simulink model "DAPS_SA_MdlIdent"  (R2017a)
settings: Solver=FixedStepAuto  StartTime=0  StopTime=68  FixedStep=0.001  MaxStep=0.01  RelTol=1e-4
undefined symbols (not defined in the file or in its folder): mdlPara
libraries: PASL_Mechanics x4, PASL_Models x2, PASL_Tools x2, PASL_Pneumatics x2, PASL_Components x1
settings Model: Creator=MMNT  LastModifiedBy=mmnt

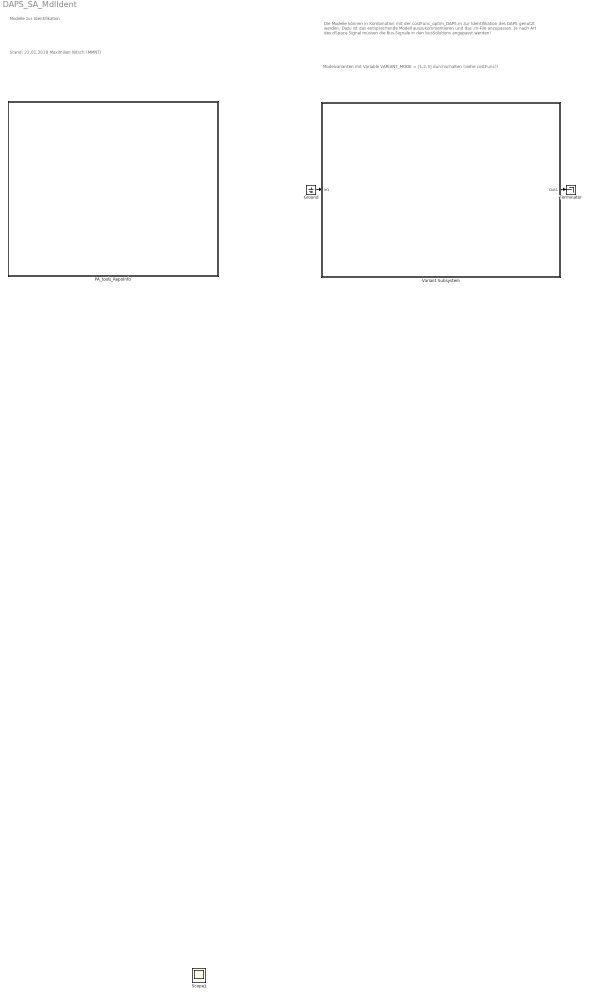
== system DAPS_SA_MdlIdent ==
  note: Modelvarianten mit Variable VARIANT_MODE = [1,2,3] durchschalten (siehe costFunc)!
  note: Die Modelle können in Kombination mit der costFunc_optim_DAPS.m
      | zur Identifikation des DAPS genutzt werden. Dazu ist das entsprechende
      | Modell auszukommentieren und das .m-File anzupassen. Je nach Art des
      | dSpace Signal müssen die Bus-Signale in den busSolutions angepasst werden!
  note: Modelle zur Identifikation
  note: Stand: 22.01.2018
      | Maximilian Nitsch (MMNT)
  Ground : Ground
  PA_tools_RepoInfo : Subsystem  Tag=RevTagSubSys  mask(cover){}
      mask help: mask for library reasons
      settings: OpenFcn=PA_setRepoInfoBlock()
      mask Help: eval(['run(strcat(''',getenv('pasl_simulink'),''',''\documentation\tools\HelpForPaslElements.m''))']);
      mask Display: text(.05,.95,'Project:\n   Rev#:  33\n   RevID: 6ffad1a574bd\n   date:  Thu Jan 25 10:31:59 2018 +0100\n\nPASL:\n   Rev#:  456\n   RevID: 2bc290b3a386\n   date:  Mon Jan 29 08:53:47 2018 +0100\n\nPATL:\n   Rev#:  74\n   RevID: 19f2c7ed23f7\n   date:  Thu Jan 25 10:02:33 2018 +0100','hor','left','ver','top')
  Terminator : Terminator
  Variant Subsystem : Subsystem  Variant=on
  Scope1 : Scope
  wires:
  Ground/1 -> Variant Subsystem/1(In1)
  Variant Subsystem/1(Out1) -> Terminator/1

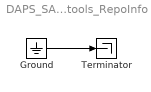
== system DAPS_SA_MdlIdent/PA_tools_RepoInfo ==
  Ground : Ground
  Terminator : Terminator
  wires:
  Ground/1 -> Terminator/1

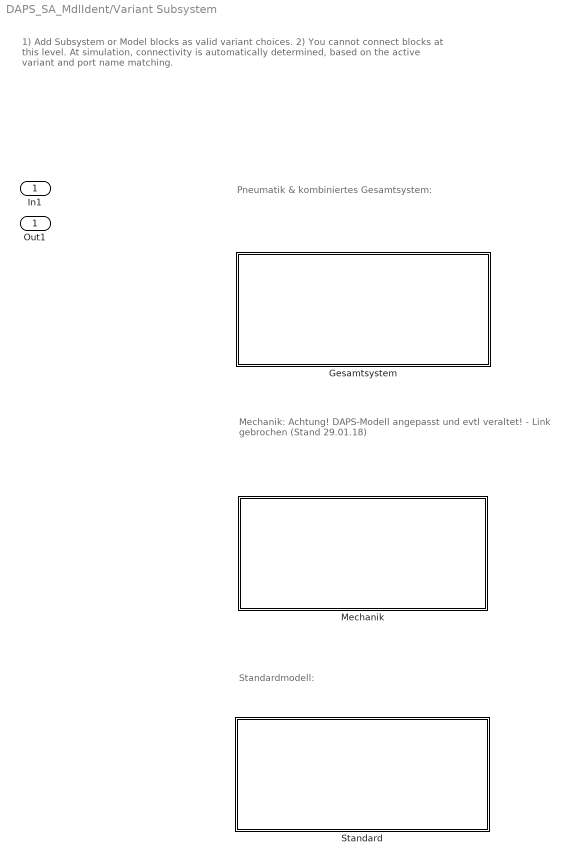
== system DAPS_SA_MdlIdent/Variant Subsystem ==
  note: 1) Add Subsystem or Model blocks as valid variant choices.
      | 2) You cannot connect blocks at this level. At simulation, connectivity is automatically
      | determined, based on the active variant and port name matching.
  note: Pneumatik & kombiniertes Gesamtsystem:
  note: Standardmodell:
  note: Mechanik:
      | Achtung! DAPS-Modell angepasst und evtl veraltet!
      | - Link gebrochen (Stand 29.01.18)
  In1 : Inport
  Gesamtsystem : Subsystem  VariantControl=VARIANT_MODE == 1
  Mechanik : Subsystem  VariantControl=VARIANT_MODE == 2
  Standard : Subsystem  VariantControl=VARIANT_MODE == 3
  Out1 : Outport

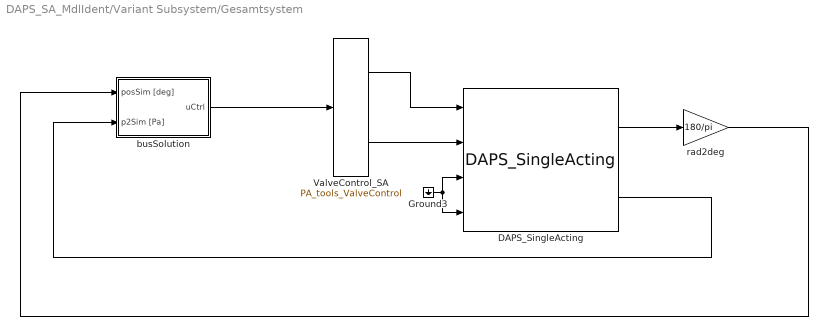
== system DAPS_SA_MdlIdent/Variant Subsystem/Gesamtsystem ==
  DAPS_SingleActing : PASL_Models/DAPS_SingleActing  mdlPara=mdlPara
      settings: SourceProductName=PASL
  Ground3 : Ground
  ValveControl_SA : PASL_Tools/PA_tools_ValveControl
      settings: SourceProductName=PASL
  busSolution : Subsystem  VariantControl=busVariant
  rad2deg : Gain  Gain=180/pi
  wires:
  rad2deg/1 -> busSolution/1(posSim [deg])
  DAPS_SingleActing/1 -> rad2deg/1
  DAPS_SingleActing/2 -> busSolution/2(p2Sim [Pa])
  Ground3/1 -> DAPS_SingleActing/3, DAPS_SingleActing/4
  busSolution/1(uCtrl) -> ValveControl_SA/1
  ValveControl_SA/2 -> DAPS_SingleActing/2
  ValveControl_SA/1 -> DAPS_SingleActing/1

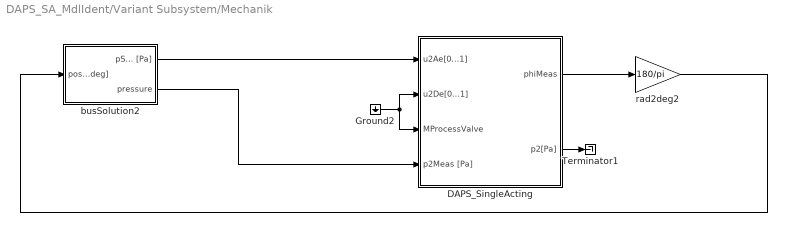
== system DAPS_SA_MdlIdent/Variant Subsystem/Mechanik ==
  DAPS_SingleActing : Subsystem  AncestorBlock=PASL_Models/DAPS_SingleActing  mask(Einfachwirkender DAPS){mdlPara=mdlPara}
      mask prompts: mdlPara "Name of the parameters struct:"
      mask help:
      | Dieses Subsystem beinhaltet das Modell eines
      | einfachwirkenden DAPSs.
      |
      | Zur Initialisierung des Systems kann entweder
      | a) ein vorhandener Parametersatz geladen werden
      | oder
      | b) ein default Datensatz generiert werden.
      | Dabei werden die Daten des DAPS abgefragt
      | und alle aus der Konstruktion bekannten
      | Parameter entsprechend berechnet.
      |
      |
      |
      | 18.01.2018, Maximilian Nitsch (MMNT)
      mask DialogControl Control2 Prompt: Parametersatz laden
      mask DialogControl Control2 Callback:
      | %% Modellparameter laden %%%%%%%%%%%%%%%%%%%%%%%%%%%%%%%%%%%%%%%%%%%%%%%%%%
      | 
      | % get mask parameters
      | maskval = get_param(gcb,'MaskValues');
      | structName = maskval{1};
      | 
      | % load parameters
      | assignin('base',structName,...
      | 	aux_loadMdlPara('DAPS','mdlPara_DAPS-0053-090-RS4-F0507_PSA-01-RT-O-171018-0649.mat')...
      | 	);
      | 
      | % clear section
      | clear maskval structName
      mask DialogControl Control3 Prompt: Parametersatz generieren
      mask DialogControl Control3 Callback:
      | %% Modellparameter laden %%%%%%%%%%%%%%%%%%%%%%%%%%%%%%%%%%%%%%%%%%%%%%%%%%
      | 
      | % get mask parameters
      | maskval = get_param(gcb,'MaskValues');
      | structName = maskval{1};
      | 
      | % load parameters
      | assignin('base',structName,aux_initMdlParaDAPS_SA());
      | 
      | % clear section
      | clear maskval structName
      mask Display:
      | image('DAPS_SingleActing.jpg')
      | 
      | color('black')
      | port_label('input',1,'u2Ae [0...1]')
      | port_label('input',2,'u2De [0...1]')
      | port_label('input',3,'MProcessValve')
      | port_label('input',4,'p2 [Pa] (optional)')
      | 
      | port_label('output',1,'phiMeas [rad]')
      | port_label('output',2,'p2Sim [Pa]')
  Ground2 : Ground
  Terminator1 : Terminator
  busSolution2 : Subsystem  VariantControl=busVariant
  rad2deg2 : Gain  Gain=180/pi
  wires:
  busSolution2/2(pressure) -> DAPS_SingleActing/4(p2Meas [Pa])
  rad2deg2/1 -> busSolution2/1(posSim [deg])
  busSolution2/1(pSoll [Pa]) -> DAPS_SingleActing/1(u2Ae[0...1])
  Ground2/1 -> DAPS_SingleActing/3("MProcessValve "), DAPS_SingleActing/2(u2De[0...1])
  DAPS_SingleActing/2(p2[Pa]) -> Terminator1/1
  DAPS_SingleActing/1("phiMeas ") -> rad2deg2/1

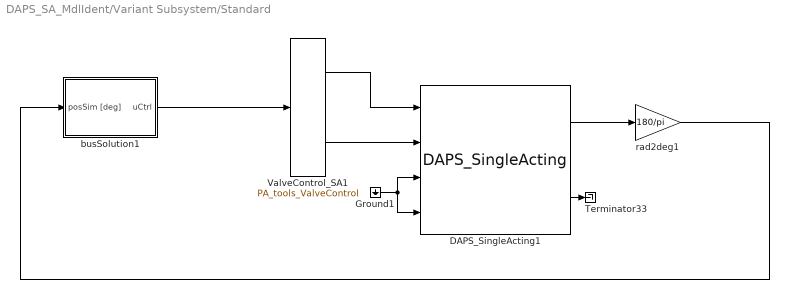
== system DAPS_SA_MdlIdent/Variant Subsystem/Standard ==
  DAPS_SingleActing1 : PASL_Models/DAPS_SingleActing  mdlPara=mdlPara
      settings: SourceProductName=PASL
  Ground1 : Ground
  Terminator33 : Terminator
  ValveControl_SA1 : PASL_Tools/PA_tools_ValveControl
      settings: SourceProductName=PASL
  busSolution1 : Subsystem  VariantControl=busVariant
  rad2deg1 : Gain  Gain=180/pi
  wires:
  rad2deg1/1 -> busSolution1/1(posSim [deg])
  Ground1/1 -> DAPS_SingleActing1/4, DAPS_SingleActing1/3
  ValveControl_SA1/2 -> DAPS_SingleActing1/2
  ValveControl_SA1/1 -> DAPS_SingleActing1/1
  busSolution1/1(uCtrl) -> ValveControl_SA1/1
  DAPS_SingleActing1/1 -> rad2deg1/1
  DAPS_SingleActing1/2 -> Terminator33/1

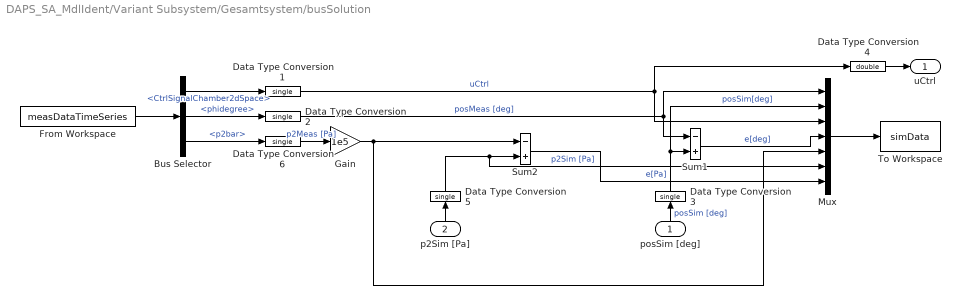
== system DAPS_SA_MdlIdent/Variant Subsystem/Gesamtsystem/busSolution ==
  posSim [deg] : Inport
  p2Sim [Pa] : Inport  Port=2
  Bus Selector : BusSelector  OutputSignals=CtrlSignalChamber2dSpace,phidegree,p2bar
  Data Type Conversion{1..3,5..6} (5 alike) : DataTypeConversion  OutDataTypeStr=single
  Data Type Conversion4 : DataTypeConversion  OutDataTypeStr=double
  From Workspace : FromWorkspace  VariableName=measDataTimeSeries  OutDataTypeStr=Bus: busMeasData  SampleTime=0  OutputAfterFinalValue=Setting to zero
  Gain : Gain  Gain=1e5
  Mux : Mux  Inputs=7
  Sum1 : Sum  Inputs=-+
  Sum2 : Sum  Inputs=-+
  To Workspace : ToWorkspace  VariableName=simData  SaveFormat=Structure With Time  SampleTime=-1
  uCtrl : Outport
  wires:
  Data Type Conversion4/1 -> uCtrl/1
  Data Type Conversion3/1 -> Mux/2, Sum1/2  "posSim[deg]"
  Data Type Conversion2/1 -> Sum1/1, Mux/1  "posMeas [deg]"
  Data Type Conversion1/1 -> Data Type Conversion4/1, Mux/3  "uCtrl"
  Mux/1 -> To Workspace/1
  Sum1/1 -> Mux/4  "e[deg]"
  posSim [deg]/1 -> Data Type Conversion3/1  "posSim [deg]"
  From Workspace/1 -> Bus Selector/1
  Bus Selector/1 -> Data Type Conversion1/1  "<CtrlSignalChamber2dSpace>"
  Bus Selector/2 -> Data Type Conversion2/1  "<phidegree>"
  Bus Selector/3 -> Data Type Conversion6/1  "<p2bar>"
  p2Sim [Pa]/1 -> Data Type Conversion5/1
  Data Type Conversion6/1 -> Gain/1  "p2Meas [Pa]"
  Data Type Conversion5/1 -> Mux/6, Sum2/2  "p2Sim [Pa]"
  Sum2/1 -> Mux/7  "e[Pa]"
  Gain/1 -> Sum2/1, Mux/5

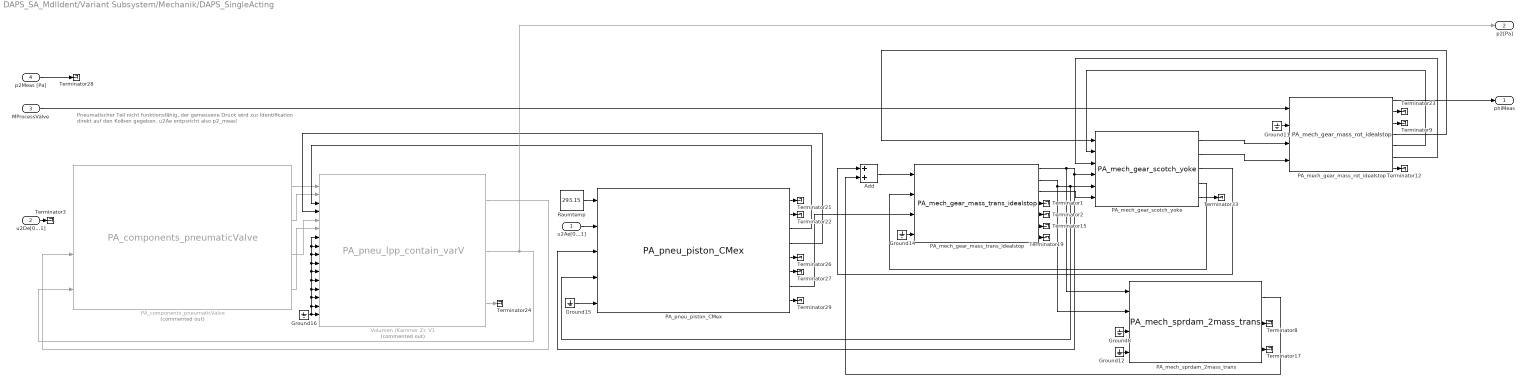
== system DAPS_SA_MdlIdent/Variant Subsystem/Mechanik/DAPS_SingleActing ==
  note: Pneumatischer Teil nicht funktionsfähig, der gemessene Druck wird zur Identifikation
      | direkt auf den Kolben gegeben. u2Ae entpsricht also p2_meas!
  u2Ae[0...1] : Inport
  u2De[0...1] : Inport  Port=2
  "MProcessValve " : Inport  Port=3
  p2Meas [Pa] : Inport  Port=4
  Add : Sum
  Ground{8,11..12,14..16} (6 alike) : Ground
  PA_components_pneumaticValve : PASL_Components/PA_components_pneumaticValve  Commented=on  b=mdlPara.b  C=mdlPara.C2  pv=mdlPara.pv  pu=mdlPara.pu  Tu=mdlPara.Tu  R=mdlPara.R  n=mdlPara.n  smoothFact=mdlPara.smoothFac
      settings: SourceProductName=PASL
  PA_mech_gear_mass_rot_idealstop : PASL_Mechanics/Gear Elements/PA_mech_gear_mass_rot_idealstop  Tag=RB_mech_gear_mass_rot_idealstop  phiinit=mdlPara.Phi0  phidotinit=mdlPara.Phidot0  J=mdlPara.Inertia  drot1=mdlPara.PinionViscFri  drot2=0.0  drot3=0.0  phidotstri=mdlPara.PinionStribeckVel  Mstick=mdlPara.PinionMstick  Mslip=mdlPara.PinionMcoulomb  phimin=mdlPara.PhiMin  phimax=mdlPara.PhiMax
      settings: SourceProductName=PASL
  PA_mech_gear_mass_trans_idealstop : PASL_Mechanics/Gear Elements/PA_mech_gear_mass_trans_idealstop  Tag=RB_mech_gear_mass_rot_idealstop  xinit=mdlPara.z0  xdotinit=mdlPara.v0  m=mdlPara.mass  dtrans1=mdlPara.viscFriCoeff1  dtrans2=0.0  dtrans3=0.0  xdotstri=mdlPara.stribeckVel  Fstick=mdlPara.Fstick  Fslip=mdlPara.Fcoulomb  xmin=mdlPara.zMin  xmax=mdlPara.zMax
      settings: SourceProductName=PASL
  PA_mech_gear_scotch_yoke : PASL_Mechanics/Gear Elements/PA_mech_gear_scotch_yoke  Tag=PA_mech_gear_rack  e1=mdlPara.e1  e2=mdlPara.e2  lot=0  xMin=mdlPara.xMin  dx0=0  cintern=mdlPara.cx  dintern=mdlPara.dx  Fdmax=200  eta=1  etamode=mode 2: exact
      settings: SourceProductName=PASL
  PA_mech_sprdam_2mass_trans : PASL_Mechanics/Spring and Damping Elements/PA_mech_sprdam_2mass_trans  Tag=PA_mech_sprdam_2mass_trans  ctrans=mdlPara.c  dtrans=mdlPara.d  x0=mdlPara.zfZero  lot=mdlPara.transLot
      settings: SourceProductName=PASL
  PA_pneu_piston_CMex : PASL_Pneumatics/Pistons/PA_pneu_piston_CMex  d_out=mdlPara.dOut  d_in=mdlPara.dIn  p0=mdlPara.pu  x_0=mdlPara.initChamberLength
      settings: SourceProductName=PASL
  Raumtemp : Constant  Value=293.15
  Terminator{1..3,8..9,12,15,17,19,21..24,26..29,33} (18 alike) : Terminator
  Volumen (Kammer 2): V1 : PASL_Pneumatics/Volumes/PA_pneu_lpp_contain_varV  Commented=on  p0=mdlPara.p02  T0=mdlPara.Tu  V0=mdlPara.V0  K=mdlPara.heatExCoeff  A=mdlPara.heatExArea  Tw=mdlPara.Tu  R=mdlPara.R  kappa=mdlPara.n  temp_effects=without temperature effects
      settings: SourceProductName=PASL
  "phiMeas " : Outport
  p2[Pa] : Outport  Port=2
  wires:
  p2Meas [Pa]/1 -> Terminator28/1
  PA_mech_gear_mass_trans_idealstop/2 -> PA_pneu_piston_CMex/4, PA_mech_gear_scotch_yoke/5, PA_mech_sprdam_2mass_trans/2
  PA_mech_gear_mass_trans_idealstop/1 -> PA_pneu_piston_CMex/3, PA_mech_gear_scotch_yoke/4, PA_mech_sprdam_2mass_trans/1
  PA_mech_gear_scotch_yoke/4 -> PA_mech_gear_mass_trans_idealstop/2
  PA_mech_gear_mass_trans_idealstop/6 -> Terminator15/1
  PA_mech_gear_mass_trans_idealstop/7 -> Terminator19/1
  PA_mech_gear_scotch_yoke/3 -> Add/1
  PA_mech_gear_mass_rot_idealstop/7 -> Terminator12/1
  PA_mech_gear_mass_rot_idealstop/3 -> Terminator9/1
  PA_mech_sprdam_2mass_trans/1 -> Add/2
  PA_mech_gear_mass_rot_idealstop/6 -> PA_mech_gear_scotch_yoke/3
  PA_mech_sprdam_2mass_trans/3 -> Terminator17/1
  PA_mech_gear_scotch_yoke/2 -> PA_mech_gear_mass_rot_idealstop/4
  Ground11/1 -> PA_mech_gear_mass_rot_idealstop/2
  PA_mech_gear_mass_rot_idealstop/1 -> "phiMeas "/1
  PA_mech_sprdam_2mass_trans/2 -> Terminator8/1
  PA_mech_gear_mass_rot_idealstop/5 -> PA_mech_gear_scotch_yoke/2
  Add/1 -> PA_mech_gear_mass_trans_idealstop/1
  PA_mech_gear_mass_rot_idealstop/2 -> Terminator23/1
  PA_mech_gear_mass_rot_idealstop/4 -> PA_mech_gear_scotch_yoke/1
  Ground12/1 -> PA_mech_sprdam_2mass_trans/4
  PA_mech_gear_scotch_yoke/1 -> PA_mech_gear_mass_rot_idealstop/3
  Ground8/1 -> PA_mech_sprdam_2mass_trans/3
  Ground14/1 -> PA_mech_gear_mass_trans_idealstop/4
  PA_pneu_piston_CMex/7 -> PA_mech_gear_mass_trans_idealstop/3
  Ground15/1 -> PA_pneu_piston_CMex/5
  PA_pneu_piston_CMex/1 -> Terminator21/1
  PA_pneu_piston_CMex/2 -> Terminator22/1
  PA_pneu_piston_CMex/5 -> Terminator26/1
  PA_pneu_piston_CMex/6 -> Terminator27/1
  PA_pneu_piston_CMex/8 -> Terminator29/1
  PA_mech_gear_scotch_yoke/5 -> Terminator33/1
  PA_components_pneumaticValve/1 -> Volumen (Kammer 2): V1/1
  PA_components_pneumaticValve/2 -> Volumen (Kammer 2): V1/2
  PA_components_pneumaticValve/3 -> Volumen (Kammer 2): V1/5
  PA_components_pneumaticValve/4 -> Volumen (Kammer 2): V1/6
  Ground16/1 -> Volumen (Kammer 2): V1/7, Volumen (Kammer 2): V1/8, Volumen (Kammer 2): V1/9, Volumen (Kammer 2): V1/10, Volumen (Kammer 2): V1/11, Volumen (Kammer 2): V1/12, Volumen (Kammer 2): V1/13, Volumen (Kammer 2): V1/14, Volumen (Kammer 2): V1/15, Volumen (Kammer 2): V1/16
  PA_pneu_piston_CMex/3 -> Volumen (Kammer 2): V1/3
  PA_pneu_piston_CMex/4 -> Volumen (Kammer 2): V1/4
  Volumen (Kammer 2): V1/2 -> p2[Pa]/1, PA_components_pneumaticValve/4
  Volumen (Kammer 2): V1/1 -> PA_components_pneumaticValve/3
  Volumen (Kammer 2): V1/3 -> Terminator24/1
  "MProcessValve "/1 -> PA_mech_gear_mass_rot_idealstop/1
  PA_mech_gear_mass_trans_idealstop/3 -> PA_mech_gear_scotch_yoke/6
  PA_mech_gear_mass_trans_idealstop/4 -> Terminator1/1
  PA_mech_gear_mass_trans_idealstop/5 -> Terminator2/1
  Raumtemp/1 -> PA_pneu_piston_CMex/1
  u2Ae[0...1]/1 -> PA_pneu_piston_CMex/2
  u2De[0...1]/1 -> Terminator3/1

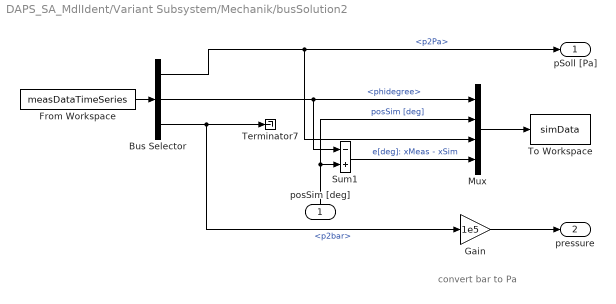
== system DAPS_SA_MdlIdent/Variant Subsystem/Mechanik/busSolution2 ==
  note: convert bar to Pa
  posSim [deg] : Inport
  Bus Selector : BusSelector  OutputSignals=p2Pa,phidegree,p2bar
  From Workspace : FromWorkspace  VariableName=measDataTimeSeries  OutDataTypeStr=Bus: busMeasData  SampleTime=0  OutputAfterFinalValue=Setting to zero
  Gain : Gain  Gain=1e5
  Mux : Mux
  Sum1 : Sum  Inputs=-+
  Terminator7 : Terminator
  To Workspace : ToWorkspace  VariableName=simData  SaveFormat=Structure With Time  SampleTime=-1
  pSoll [Pa] : Outport
  pressure : Outport  Port=2
  wires:
  Mux/1 -> To Workspace/1
  Sum1/1 -> Mux/4  "e[deg]: xMeas - xSim"
  posSim [deg]/1 -> Mux/2, Sum1/2  "posSim [deg]"
  From Workspace/1 -> Bus Selector/1
  Bus Selector/2 -> Mux/1, Sum1/1  "<phidegree>"
  Bus Selector/1 -> pSoll [Pa]/1, Mux/3  "<p2Pa>"
  Bus Selector/3 -> Gain/1, Terminator7/1  "<p2bar>"
  Gain/1 -> pressure/1

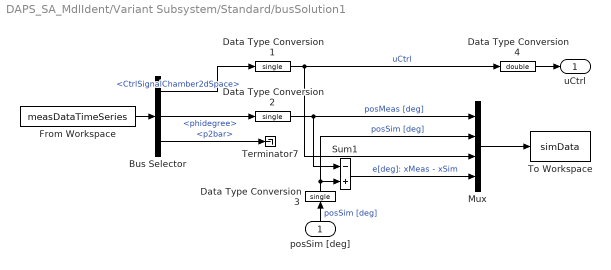
== system DAPS_SA_MdlIdent/Variant Subsystem/Standard/busSolution1 ==
  posSim [deg] : Inport
  Bus Selector : BusSelector  OutputSignals=CtrlSignalChamber2dSpace,phidegree,p2bar
  Data Type Conversion1 : DataTypeConversion  OutDataTypeStr=single
  Data Type Conversion2 : DataTypeConversion  OutDataTypeStr=single
  Data Type Conversion3 : DataTypeConversion  OutDataTypeStr=single
  Data Type Conversion4 : DataTypeConversion  OutDataTypeStr=double
  From Workspace : FromWorkspace  VariableName=measDataTimeSeries  OutDataTypeStr=Bus: busMeasData  SampleTime=0  OutputAfterFinalValue=Setting to zero
  Mux : Mux
  Sum1 : Sum  Inputs=-+
  Terminator7 : Terminator
  To Workspace : ToWorkspace  VariableName=simData  SaveFormat=Structure With Time  SampleTime=-1
  uCtrl : Outport
  wires:
  Data Type Conversion4/1 -> uCtrl/1
  Data Type Conversion3/1 -> Mux/2, Sum1/2  "posSim [deg]"
  Data Type Conversion2/1 -> Mux/1, Sum1/1  "posMeas [deg]"
  Data Type Conversion1/1 -> Mux/3, Data Type Conversion4/1  "uCtrl"
  Mux/1 -> To Workspace/1
  Sum1/1 -> Mux/4  "e[deg]: xMeas - xSim"
  posSim [deg]/1 -> Data Type Conversion3/1  "posSim [deg]"
  From Workspace/1 -> Bus Selector/1
  Bus Selector/1 -> Data Type Conversion1/1  "<CtrlSignalChamber2dSpace>"
  Bus Selector/2 -> Data Type Conversion2/1  "<phidegree>"
  Bus Selector/3 -> Terminator7/1  "<p2bar>"
